simulink model "Battery_modeling_01"  (R2023a)
settings: Solver=VariableStepAuto  StartTime=0.0  StopTime=1800  RelTol=1e-3
undefined symbols (not defined in the file): Ion, Lithium
libraries: spsBatteryLib x24, spsCurrentMeasurementLib x1, spsSeriesRLCBranchLib x1, spsVoltageMeasurementLib x1, sps_lib x1

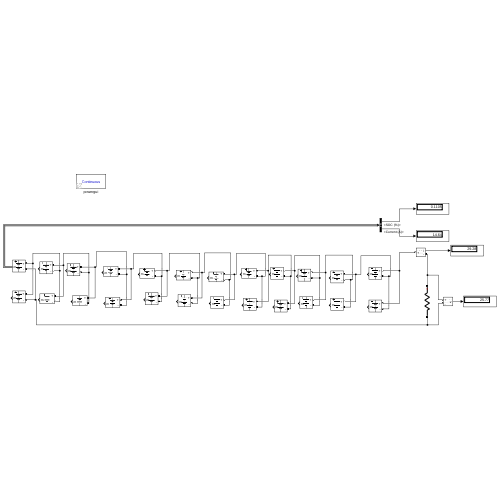
[thumbnail: Simulink's stored preview of the top-level diagram]
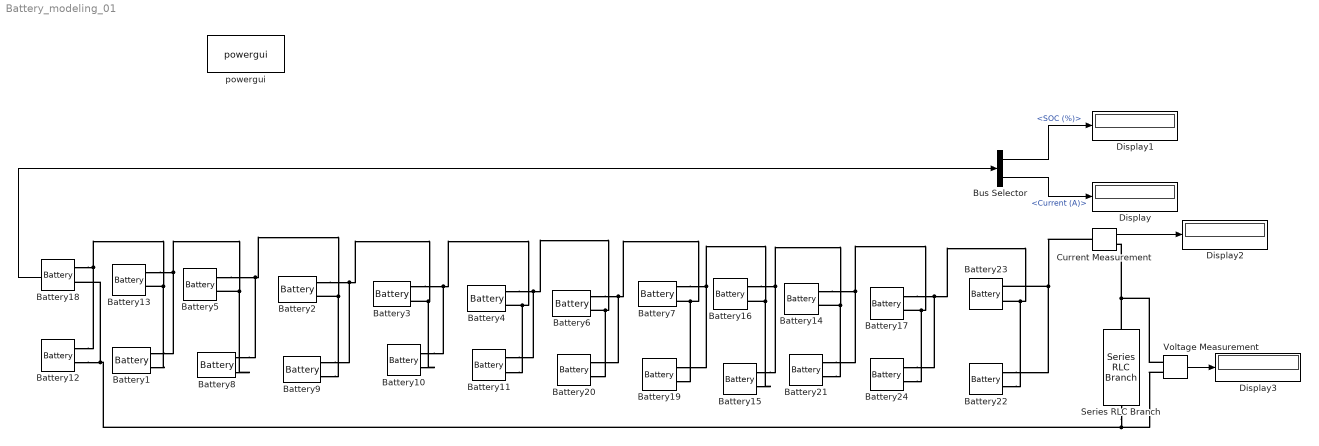
== system Battery_modeling_01 ==
  Battery{1..24} (24 alike) : spsBatteryLib/Battery  BatType=Lithium-Ion  ShowTempParam=off  ThermalPreset=no  ShowAgeParam=off  NomV=3.7  NomQ=12.5  SOC=100  Batt_Tr=30  PresetModel=on  MaxQ=12.5  MinV=2.775  FullV=4.3068  Dis_rate=5.4348  R=0.00296  Normal_OP=11.3043  expZone="[3.9974     0.61413]"  current=[6.5 13 32.5]  Units=Time  Tci=20  NomT=20  T2=-30  MaxQ2=4.8  FullV2=7.1  Normal_OP2=5.655  expZone2="[6.58           1]"  Rca=0.6  ti=2000  Dp=0  Neq0=0  Tsim=1e6  Ta1=25  Qeol=5.4*0.9  Reol=0.013333*1.2  Char_age=[2.3478, 3]  Dis_age=[2.3478, 10]  N1=1500  N2=10500  N3=1000  N4=1400  Ta2=45  N5=950
  Bus Selector : BusSelector  OutputSignals=SOC (%),Current (A)
  Current Measurement : spsCurrentMeasurementLib/Current Measurement  PhasorSimulation=off  OutputType=Complex  PSBequivalent=0
  Display{,1..3} (4 alike) : Display
  Series RLC Branch : spsSeriesRLCBranchLib/Series RLC Branch  LConnTagsString=__new0  RConnTagsString=__new0  BranchType=R  Resistance=0.88  Inductance=1e-3  SetiL0=off  InitialCurrent=0  Capacitance=1e-6  Setx0=off  InitialVoltage=0  Measurements=None
  Voltage Measurement : spsVoltageMeasurementLib/Voltage Measurement  PhasorSimulation=off  OutputType=Complex  PSBequivalent=0
  powergui : sps_lib/powergui  Priority=1  SimulationMode=Continuous  SampleTime=50e-6  frequency=60  Iterations=50  frequencyindice=0  Pbase=100e6  ErrMax=1e-4  UnitsV=kV  UnitsW=MW  buscounter=0  FunctionMessages=off  echomessages=off  EnableUseOfTLC=off  CurrentSourceSwitches=off  DisableSnubberDevices=off  DisableRonSwitches=off  DisableVfSwitches=off  DisplayEquations=off  AutomaticDiscreteSolvers=off  SolverType=Tustin/Backward Euler (TBE)  Interpol=off  ExternalGateDelay=off  methode=off  Ts=100  x0status=blocks  SPID=on  SwTol=0  HookPort=off  NonlinearTolerance=1e-4  nMaxIteration=100  ContinueOnMaxIteration=off  RestoreLinks=warning  ResistiveCurrentMeasurement=off  Frange=[0:2:500]  Ylog=off  Xlog=on  ShowGrid=off  save=off  variable=ZData  structure=0  ZoomFFT=off  StartTime=0.0  cycles=1  DisplayStyle=1  fundamental=60  FreqAxis=off  MaxFrequency=1000  frequencyindicesteady=1  RmsSteady=1  display=off
  wires:
  Battery18/1 -> Bus Selector/1
  Bus Selector/1 -> Display1/1  "<SOC (%)>"
  Bus Selector/2 -> Display/1  "<Current (A)>"
  Voltage Measurement/1 -> Display3/1
  Current Measurement/1 -> Display2/1
  connections:
  Battery18/LConn1 -- Battery12/LConn1 -- Battery1/LConn2 -- Battery13/LConn2
  Battery13/LConn1 -- Battery8/LConn2 -- Battery5/LConn2 -- Battery1/LConn1
  Battery5/LConn1 -- Battery8/LConn1 -- Battery2/LConn2 -- Battery9/LConn2
  Battery2/LConn1 -- Battery9/LConn1 -- Battery10/LConn2 -- Battery3/LConn2
  Battery3/LConn1 -- Battery10/LConn1 -- Battery11/LConn2 -- Battery4/LConn2
  Battery4/LConn1 -- Battery11/LConn1 -- Battery20/LConn2 -- Battery6/LConn2
  Battery6/LConn1 -- Battery20/LConn1 -- Battery19/LConn2 -- Battery7/LConn2
  Battery7/LConn1 -- Battery19/LConn1 -- Battery15/LConn2 -- Battery16/LConn2
  Battery16/LConn1 -- Battery21/LConn2 -- Battery14/LConn2 -- Battery15/LConn1
  Battery14/LConn1 -- Battery24/LConn2 -- Battery17/LConn2 -- Battery21/LConn1
  Battery17/LConn1 -- Battery24/LConn1 -- Battery22/LConn2 -- Battery23/LConn2
  Battery12/LConn2 -- Voltage Measurement/LConn2 -- Series RLC Branch/RConn1 -- Battery18/LConn2
  Battery22/LConn1 -- Current Measurement/LConn1 -- Battery23/LConn1
  Series RLC Branch/LConn1 -- Voltage Measurement/LConn1 -- Current Measurement/RConn1
